simulink model "IP_Raynolds_IPLT"  (R2022a)
settings: Solver=FixedStepAuto  StartTime=0.0  StopTime=30  FixedStep=0.0160  RelTol=1e-3
values from neighbouring files (symbols this model uses):
  c = 1.304    [Param_IP.m]
  G = 0.83    [Param_IP.m]
  g = 9.8    [Param_IP.m]
  G_c = 0.088    [Param_IP.m]
  Gain_Noise = 1.405    [Param_IP.m]
  h = 1.0380    (= 1.038)    [Param_IP.m]
  J = 1.15*m*(h^2)    (= 111.515454)    [Param_IP.m]
  Kd = 320.4    [Param_IP.m]
  Kp = 1114    [Param_IP.m]
  m = 90    [Param_IP.m]
  t_d = 0.060    (= 0.06)    [Param_IP.m]
settings Model: Creator=youssef  LastModifiedBy=youss
settings SolverCC: AlgebraicLoopSolver=TrustRegion
settings DataIOCC: SaveOutput=off  SignalLogging=off  DSMLogging=off  SaveTime=off  ReturnWorkspaceOutputs=off
settings OptimizationCC: ZeroExternalMemoryAtStartup=off  ZeroInternalMemoryAtStartup=off
settings DebuggingCC: UnconnectedInputMsg=warning  UnconnectedOutputMsg=warning  UnconnectedLineMsg=warning  SFMachineParentedDataDiag=warning  ArithmeticOperatorsInVariantConditions=warning
settings SFSimCC: CustomCodeUndefinedFunction=UseInterfaceOnly  SimTargetLang=C++
settings RTWCC: GenCodeOnly=on  TargetLang=C++
settings CodeAppCC: MaxIdLength=40
settings GRTTargetCC: TargetLangStandard=C++03 (ISO)  CodeReplacementLibrary=GNU C99 extensions  MatFileLogging=off  CodeInterfacePackaging=C++ class

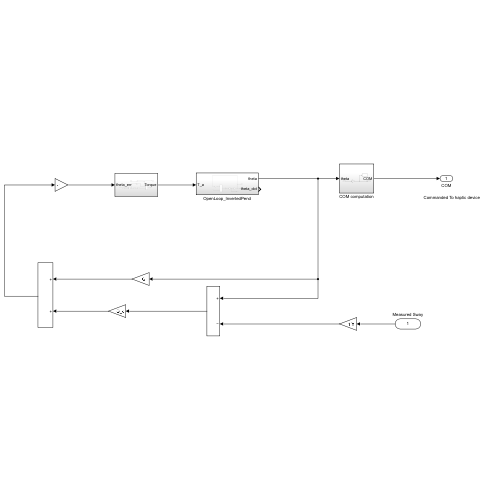
[thumbnail: Simulink's stored preview of the top-level diagram]
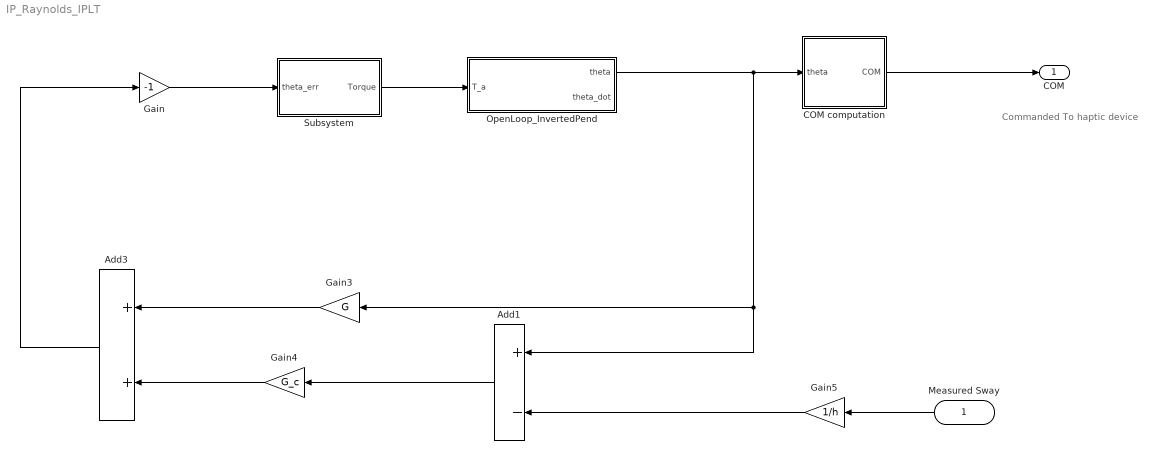
== system IP_Raynolds_IPLT ==
  note: Commanded To haptic device
  Measured Sway : Inport
  Add1 : Sum  Inputs=+-
  Add3 : Sum
  COM computation : Subsystem
  Gain : Gain  Gain=-1
  Gain3 : Gain  Gain=G
  Gain4 : Gain  Gain=G_c
  Gain5 : Gain  Gain=1/h
  OpenLoop_InvertedPend : Subsystem
  Subsystem : Subsystem
  COM : Outport  VectorParamsAs1DForOutWhenUnconnected=off
  wires:
  Gain5/1 -> Add1/2
  Gain/1 -> Subsystem/1(theta_err)
  Subsystem/1(Torque) -> OpenLoop_InvertedPend/1(T_a)
  Add1/1 -> Gain4/1
  Gain4/1 -> Add3/2
  Gain3/1 -> Add3/1
  OpenLoop_InvertedPend/1(theta) -> Add1/1, Gain3/1, COM computation/1(theta)
  Add3/1 -> Gain/1
  COM computation/1(COM) -> COM/1
  Measured Sway/1 -> Gain5/1

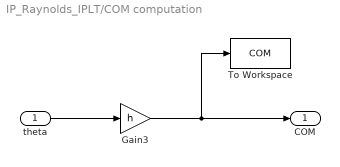
== system IP_Raynolds_IPLT/COM computation ==
  theta : Inport
  Gain3 : Gain  Gain=h
  To Workspace : ToWorkspace  VariableName=COM  SaveFormat=Timeseries  SampleTime=-1
  COM : Outport  VectorParamsAs1DForOutWhenUnconnected=off
  wires:
  theta/1 -> Gain3/1
  Gain3/1 -> To Workspace/1, COM/1

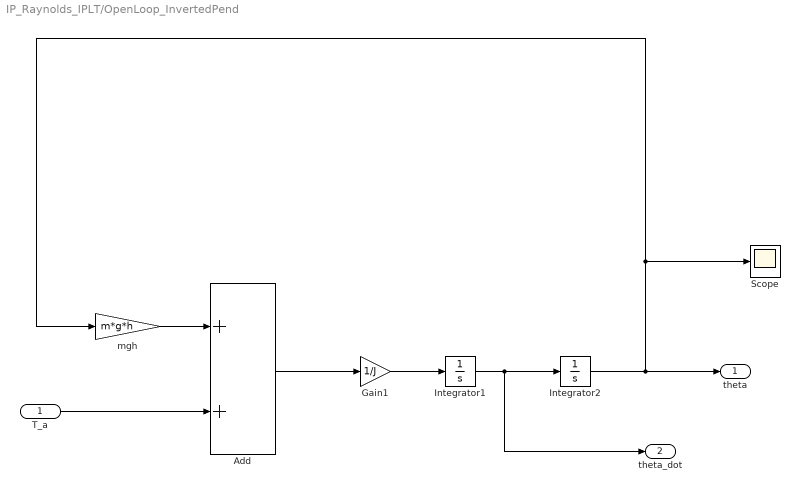
== system IP_Raynolds_IPLT/OpenLoop_InvertedPend ==
  T_a : Inport
  Add : Sum
  Gain1 : Gain  Gain=1/J
  Integrator1 : Integrator
  Integrator2 : Integrator
  Scope : Scope
  mgh : Gain  Gain=m*g*h
  theta : Outport  VectorParamsAs1DForOutWhenUnconnected=off
  theta_dot : Outport  Port=2  VectorParamsAs1DForOutWhenUnconnected=off
  wires:
  Integrator2/1 -> Scope/1, mgh/1, theta/1
  Add/1 -> Gain1/1
  Integrator1/1 -> theta_dot/1, Integrator2/1
  Gain1/1 -> Integrator1/1
  mgh/1 -> Add/1
  T_a/1 -> Add/2

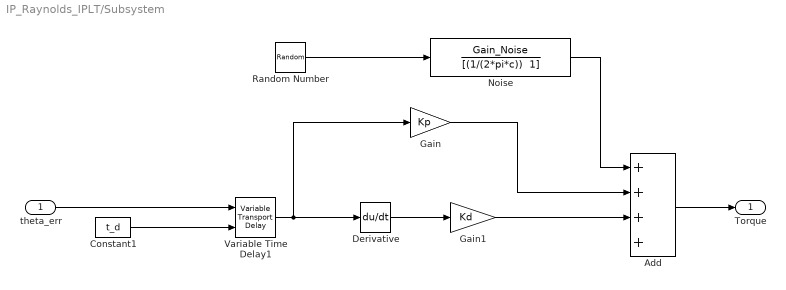
== system IP_Raynolds_IPLT/Subsystem ==
  theta_err : Inport
  Add : Sum  Inputs=++++
  Constant1 : Constant  Value=t_d
  Derivative : Derivative
  Gain : Gain  Gain=Kp
  Gain1 : Gain  Gain=Kd
  Noise : TransferFcn  Numerator=Gain_Noise  Denominator="[(1/(2*pi*c))  1]"
  Random Number : RandomNumber  SampleTime=0.16
  Variable Time Delay1 : VariableTransportDelay  MaximumDelay=10
  Torque : Outport  VectorParamsAs1DForOutWhenUnconnected=off
  wires:
  Gain/1 -> Add/2
  Random Number/1 -> Noise/1
  Derivative/1 -> Gain1/1
  Gain1/1 -> Add/3
  Add/1 -> Torque/1
  Constant1/1 -> Variable Time Delay1/2
  theta_err/1 -> Variable Time Delay1/1
  Variable Time Delay1/1 -> Gain/1, Derivative/1
  Noise/1 -> Add/1
